simulink model "wall_plumbing"  (R2017b)
settings: Solver=VariableStepAuto  StartTime=0.0  StopTime=tf  RelTol=1e-3  AbsTol=1e-3  EnableMultiTasking=on
values from neighbouring files (symbols this model uses):
  cistern_diam = 100    [plumbing_variables.m]
  cistern_inlet_diam = 2    [plumbing_variables.m]
  cistern_outlet_diam = 2    [plumbing_variables.m]
  swh_inlet_diam = 2    [plumbing_variables.m]
  swh_outlet_diam = 2    [plumbing_variables.m]
libraries: fl_lib x40, nesl_utility x28, sh_lib x10, simulink x2, SimscapeFluids_lib x1
settings Model: Creator=solan  LastModifiedBy=solan
settings SolverCC: ZeroCrossAlgorithm=Adaptive
settings DataIOCC: LimitDataPoints=on  MaxDataPoints=10000
settings OptimizationCC: LifeSpan=inf
settings DebuggingCC: AllowSymbolicDim=off  SFUnexpectedBacktrackingDiag=warning  SFNoUnconditionalDefaultTransitionDiag=warning  SFExecutionAtInitializationDiag=none
settings CodeAppCC: StateflowObjectComments=on
settings GRTTargetCC: TargetLangStandard=C89/C90 (ANSI)  GeneratePreprocessorConditionals=Disable all
settings ConfigComp: CovMetricSettings=dw  CovHtmlReporting=on  CovSaveCumulativeToWorkspaceVar=on  CovSaveSingleToWorkspaceVar=on  CovExternalEMLEnable=off  CovSFcnEnable=off
settings SimscapeCC: SimscapeLogType=all  SimscapeLogSimulationStatistics=on  SimscapeLogOpenViewer=on  SimscapeLogDataHistory=10000

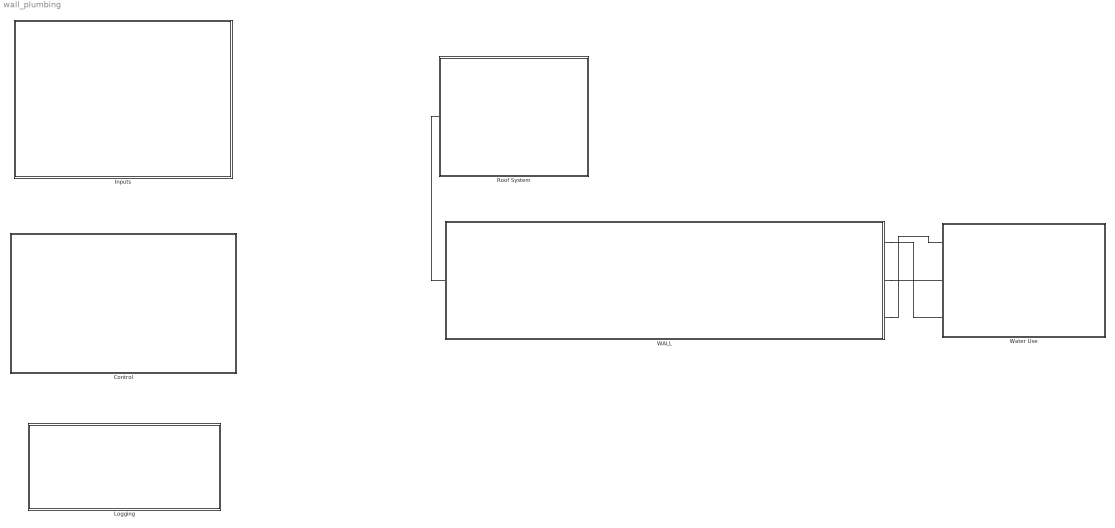
== system wall_plumbing ==
  Control : Subsystem
  Inputs : Subsystem
  Logging : Subsystem
  Roof System : Subsystem
  WALL : Subsystem
  Water Use : Subsystem
  connections:
  WALL/RConn2 -- Water Use/LConn3
  WALL/RConn1 -- Water Use/LConn2
  Roof System/LConn1 -- WALL/LConn1
  WALL/RConn3 -- Water Use/LConn1

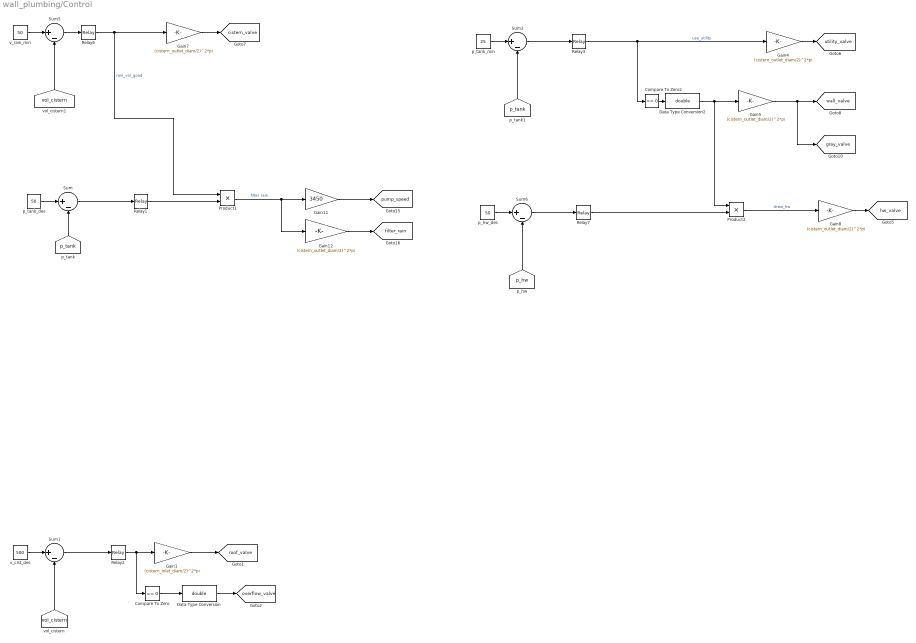
== system wall_plumbing/Control ==
  Compare To Zero : simulink/Logic and Bit Operations/Compare To Zero  relop===  OutDataTypeStr=boolean
  Compare To Zero2 : simulink/Logic and Bit Operations/Compare To Zero  relop===  OutDataTypeStr=boolean
  Data Type Conversion : DataTypeConversion  OutDataTypeStr=double
  Data Type Conversion2 : DataTypeConversion  OutDataTypeStr=double
  Gain1 : Gain  Gain=(cistern_inlet_diam/2)^2*pi
  Gain11 : Gain  Gain=3450
  Gain{4..5,7..8,12} (5 alike) : Gain  Gain=(cistern_outlet_diam/2)^2*pi
  Product1 : Product
  Product2 : Product
  Relay1 : Relay  OnSwitchValue=10  OffSwitchValue=-10
  Relay2 : Relay  OnSwitchValue=25  OffSwitchValue=-25
  Relay3 : Relay  OnSwitchValue=4  OffSwitchValue=-20
  Relay6 : Relay  OnSwitchValue=5  OffSwitchValue=-50  OnOutputValue=0  OffOutputValue=1
  Relay7 : Relay  OnSwitchValue=10  OffSwitchValue=-10
  Sum{,1..2,5..6} (5 alike) : Sum  Inputs=|+-
  p_hw_des : Constant  Value=50
  p_tank_des : Constant  Value=50
  p_tank_min : Constant  Value=25
  v_cist_des : Constant  Value=500
  v_rain_min : Constant  Value=50
  tag scope: cistern_valve=global, filter_rain=global, gray_valve=global, hw_valve=global, overflow_valve=global, pump_speed=global, roof_valve=global, utility_valve=global, wall_valve=global
  wires:
  Gain4/1 -> [utility_valve]
  Sum1/1 -> Relay2/1
  Relay3/1 -> Compare To Zero2/1, Gain4/1  "use_utility"
  Gain1/1 -> [roof_valve]
  v_cist_des/1 -> Sum1/1
  Data Type Conversion2/1 -> Product2/1, Gain5/1
  [vol_cistern] -> Sum1/2
  Sum/1 -> Relay1/1
  Gain5/1 -> [gray_valve], [wall_valve]
  [vol_cistern] -> Sum5/2
  Gain12/1 -> [filter_rain]
  [p_tank] -> Sum2/2
  Gain8/1 -> [hw_valve]
  p_tank_min/1 -> Sum2/1
  Relay1/1 -> Product1/2
  p_tank_des/1 -> Sum/1
  [p_tank] -> Sum/2
  Compare To Zero2/1 -> Data Type Conversion2/1
  Gain11/1 -> [pump_speed]
  Sum5/1 -> Relay6/1
  Sum6/1 -> Relay7/1
  Compare To Zero/1 -> Data Type Conversion/1
  p_hw_des/1 -> Sum6/1
  Gain7/1 -> [cistern_valve]
  [p_hw] -> Sum6/2
  Relay2/1 -> Compare To Zero/1, Gain1/1
  v_rain_min/1 -> Sum5/1
  Data Type Conversion/1 -> [overflow_valve]
  Relay6/1 -> Product1/1, Gain7/1  "rain_vol_good"
  Sum2/1 -> Relay3/1
  Product1/1 -> Gain12/1, Gain11/1  "filter rain"
  Relay7/1 -> Product2/2
  Product2/1 -> Gain8/1  "draw_hw"

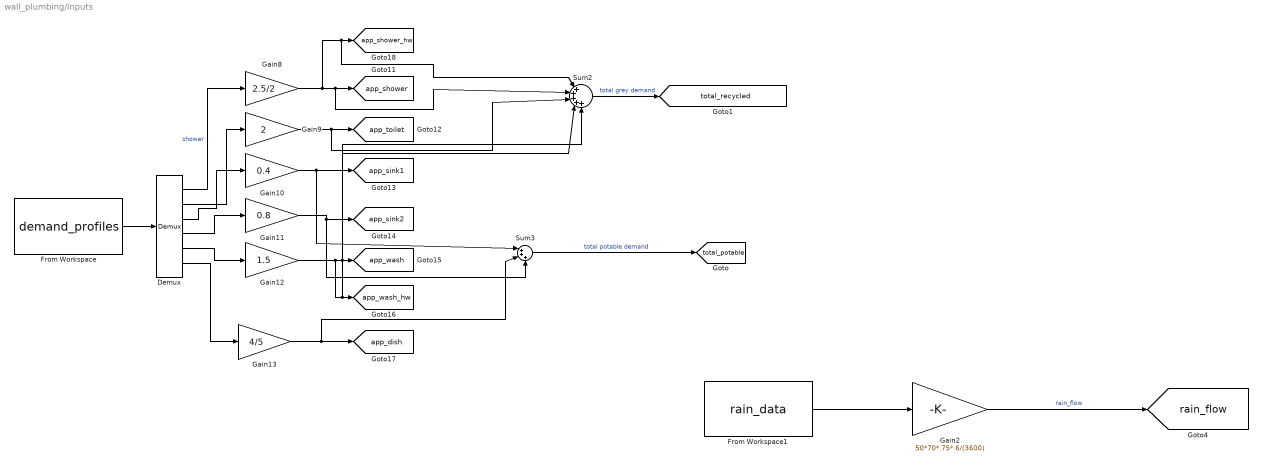
== system wall_plumbing/Inputs ==
  Demux : Demux  Outputs=6
  From Workspace : FromWorkspace  VariableName=demand_profiles  SampleTime=60
  From Workspace1 : FromWorkspace  VariableName=rain_data  SampleTime=0  Interpolate=off  OutputAfterFinalValue=Setting to zero
  Gain10 : Gain  Gain=0.4
  Gain11 : Gain  Gain=0.8
  Gain12 : Gain  Gain=1.5
  Gain13 : Gain  Gain=4/5
  Gain2 : Gain  Gain=50*70*.75*.6/(3600)
  Gain8 : Gain  Gain=2.5/2
  Gain9 : Gain  Gain=2
  Sum2 : Sum  Inputs=|+++++
  Sum3 : Sum  Inputs=|+++
  tag scope: app_dish=global, app_shower=global, app_shower_hw=global, app_sink1=global, app_sink2=global, app_toilet=global, app_wash=global, app_wash_hw=global, rain_flow=global, total_potable=global, total_recycled=global
  wires:
  From Workspace/1 -> Demux/1
  Demux/6 -> Gain13/1
  Gain2/1 -> [rain_flow]  "rain_flow"
  Gain9/1 -> Sum2/3, [app_toilet]
  Demux/4 -> Gain11/1
  Gain11/1 -> Sum3/3, [app_sink2]
  Demux/3 -> Gain10/1
  From Workspace1/1 -> Gain2/1
  Gain8/1 -> Sum2/1, [app_shower_hw], Sum2/2, [app_shower]
  Gain10/1 -> Sum3/1, [app_sink1]
  Demux/5 -> Gain12/1
  Demux/1 -> Gain8/1  "shower"
  Gain12/1 -> Sum2/5, [app_wash_hw], Sum2/4, [app_wash]
  Demux/2 -> Gain9/1
  Gain13/1 -> Sum3/2, [app_dish]
  Sum2/1 -> [total_recycled]  "total grey demand"
  Sum3/1 -> [total_potable]  "total potable demand"

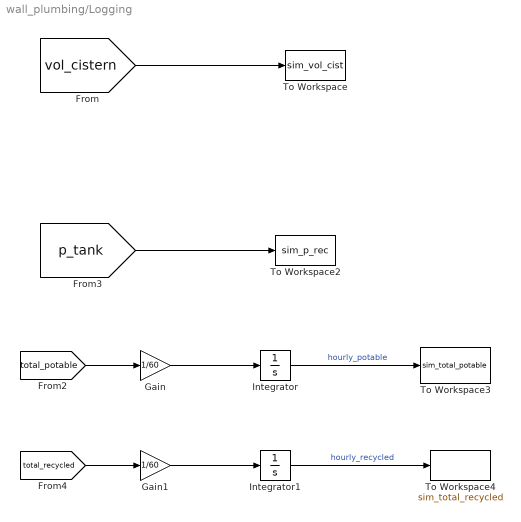
== system wall_plumbing/Logging ==
  Gain : Gain  Gain=1/60
  Gain1 : Gain  Gain=1/60
  Integrator : Integrator
  Integrator1 : Integrator
  To Workspace : ToWorkspace  VariableName=sim_vol_cist  SaveFormat=Timeseries  SampleTime=3600
  To Workspace2 : ToWorkspace  VariableName=sim_p_rec  SaveFormat=Timeseries  SampleTime=3600
  To Workspace3 : ToWorkspace  VariableName=sim_total_potable  SaveFormat=Timeseries  SampleTime=3600
  To Workspace4 : ToWorkspace  VariableName=sim_total_recycled  SaveFormat=Timeseries  SampleTime=3600
  wires:
  [vol_cistern] -> To Workspace/1
  [p_tank] -> To Workspace2/1
  [total_potable] -> Gain/1
  [total_recycled] -> Gain1/1
  Integrator1/1 -> To Workspace4/1  "hourly_recycled"
  Integrator/1 -> To Workspace3/1  "hourly_potable"
  Gain/1 -> Integrator/1
  Gain1/1 -> Integrator1/1

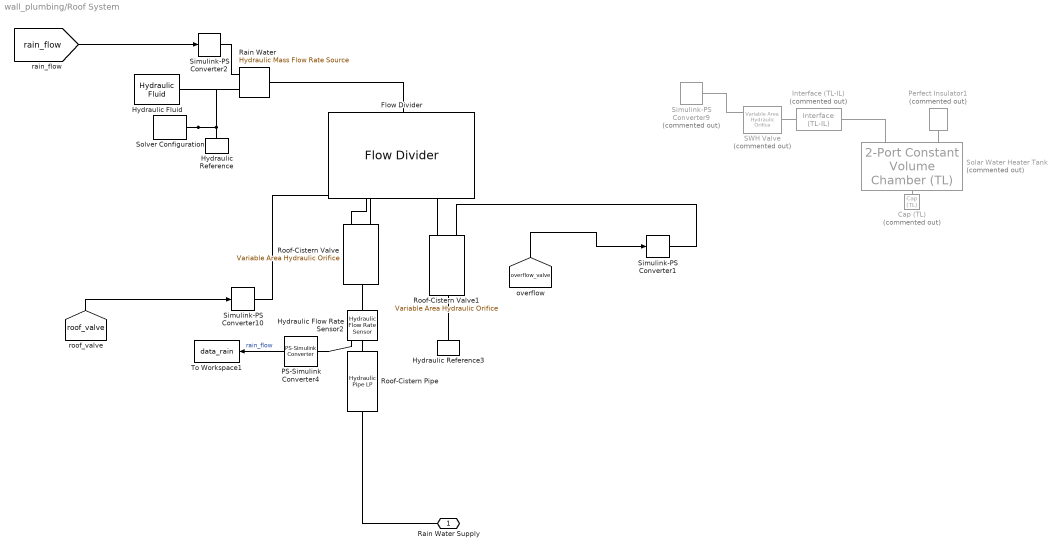
== system wall_plumbing/Roof System ==
  Cap (TL) : fl_lib/Thermal Liquid/Elements/Cap (TL)  Commented=on  p_specify=off  p_priority=None  p=0.101325 MPa  p_nominal_specify=off  p_nominal_unit=MPa  p_nominal_value=1  T_specify=off  T_priority=None  T=293.15 K  T_nominal_specify=off  T_nominal_unit=K  T_nominal_value=1
      settings: SourceProductName=Simscape  SourceProductBaseCode=SS
  Flow Divider : sh_lib/Valves/Flow Control Valves/Flow Divider  area_A=1e-4 m^2  area_B=1e-4 m^2  C_d_A=0.7  C_d_B=0.7  lam_spec=1  B_lam_A=0.999  B_lam_B=0.999  Re_cr_A=10  Re_cr_B=10  orifice_d=0.005 m  orifice_numb=4  C_d_or=0.65  init_A=0.0025 m  init_B=0.0025 m  leak_area=1e-9 m^2  lam_spec_or=1  B_lam_or_A=0.999  B_lam_or_B=0.999  Re_cr_or_A=10  Re_cr_or_B=10  area_sc=1.6e-4 m^2  stroke=0.005 m  spring_rate=1e3 N/m  damping=150 N/(m/s)  stop_coefficient=1e12 s*N/m^2
      settings: SourceProductName=Simscape Fluids  SourceProductBaseCode=SH
  Hydraulic Flow Rate Sensor2 : fl_lib/Hydraulic/Hydraulic Sensors/Hydraulic Flow Rate Sensor
      settings: SourceProductName=Simscape
  Hydraulic Fluid : sh_lib/Hydraulic Utilities/Hydraulic Fluid  DataSource=1  SelFluid=24  SysTemp=15  TrapAir=0.005  ViscDerFactor=1  range_error=2
      settings: SourceProductName=Simscape Fluids
  Hydraulic Reference : fl_lib/Hydraulic/Hydraulic Elements/Hydraulic Reference
      settings: SourceProductName=Foundation Library
  Hydraulic Reference3 : fl_lib/Hydraulic/Hydraulic Elements/Hydraulic Reference
      settings: SourceProductName=Foundation Library
  Interface (TL-IL) : SimscapeFluids_lib/Fluid Network Interfaces/Interface (TL-IL)  Commented=on  T_B=293.15 K  area=0.01 m^2
      settings: SourceProductName=Simscape Fluids  SourceProductBaseCode=SH
  PS-Simulink Converter4 : nesl_utility/PS-Simulink Converter  PhysicalDomain=network_engine_domain  SubClassName=ps_output  LeftPortType=input  RightPortType=output  PseudoPeriodic=off  Frequencies=[]  Unit=gal/s  AffineConversion=off
  Perfect Insulator1 : fl_lib/Thermal/Thermal Elements/Perfect Insulator  Commented=on  T_specify=off  T_priority=None  T=0 K  T_nominal_specify=off  T_nominal_unit=K  T_nominal_value=1
      settings: SourceProductName=Simscape
  Rain Water : fl_lib/Hydraulic/Hydraulic Sources/Hydraulic Mass Flow Rate Source
      settings: SourceProductName=Simscape  SourceProductBaseCode=SS
  Roof-Cistern Pipe : sh_lib/Low-Pressure Blocks/Hydraulic Pipe LP  cs_type=1  d_in=cistern_inlet_diam in  area=1e-4 m^2  D_h=1.12e-2 m  s_factor=64  length=roof_cistern_pipe_length ft  length_ad=1 m  roughness=15e-6 m  Re_lam=2000  Re_turb=4000  elevation_A=roof_height ft  elevation_B=cistern_inlet_height ft  g=9.80665 m/s^2  wall_type=1  pr_r_coef=2e-12 m/Pa  time_const=0.01 s  k_sh=1.4  p0=0 Pa
      settings: SourceProductName=Simscape Fluids  SourceProductBaseCode=SH
  Roof-Cistern Valve : fl_lib/Hydraulic/Hydraulic Elements/Variable Area Hydraulic Orifice  C_d=0.7  min_area=1e-12 m^2  lam_spec=1  B_lam=0.999  Re_cr=12  q_specify=off  q_priority=None  q=0.001 m^3/s  q_nominal_specify=off  q_nominal_unit=m^3/s  q_nominal_value=1  p_specify=off  p_priority=None  p=0 Pa  p_nominal_specify=off  p_nominal_unit=Pa  p_nominal_value=1
      settings: SourceProductName=Simscape  SourceProductBaseCode=SS
  Roof-Cistern Valve1 : fl_lib/Hydraulic/Hydraulic Elements/Variable Area Hydraulic Orifice  C_d=0.7  min_area=1e-12 m^2  lam_spec=1  B_lam=0.999  Re_cr=12  q_specify=off  q_priority=None  q=0.001 m^3/s  q_nominal_specify=off  q_nominal_unit=m^3/s  q_nominal_value=1  p_specify=off  p_priority=None  p=0 Pa  p_nominal_specify=off  p_nominal_unit=Pa  p_nominal_value=1
      settings: SourceProductName=Simscape  SourceProductBaseCode=SS
  SWH Valve : fl_lib/Hydraulic/Hydraulic Elements/Variable Area Hydraulic Orifice  Commented=on  C_d=0.7  min_area=1e-12 m^2  lam_spec=1  B_lam=0.999  Re_cr=12  q_specify=off  q_priority=None  q=0.001 m^3/s  q_nominal_specify=off  q_nominal_unit=m^3/s  q_nominal_value=1  p_specify=off  p_priority=None  p=0 Pa  p_nominal_specify=off  p_nominal_unit=Pa  p_nominal_value=1
      settings: SourceProductName=Simscape  SourceProductBaseCode=SS
  Simulink-PS Converter1 : nesl_utility/Simulink-PS Converter  PhysicalDomain=network_engine_domain  SubClassName=ps_input  LeftPortType=input  RightPortType=output  PseudoPeriodic=off  Frequencies=[]  NoiseDistribution=none  NoiseParameters=[]  Unit=1  AffineConversion=off  FilteringAndDerivatives=zero  SimscapeFilterOrder=1  InputFilterTimeConstant=0.001  UdotUserProvided=1
  Simulink-PS Converter10 : nesl_utility/Simulink-PS Converter  PhysicalDomain=network_engine_domain  SubClassName=ps_input  LeftPortType=input  RightPortType=output  PseudoPeriodic=off  Frequencies=[]  NoiseDistribution=none  NoiseParameters=[]  Unit=in^2  AffineConversion=off  FilteringAndDerivatives=zero  SimscapeFilterOrder=1  InputFilterTimeConstant=0.001  UdotUserProvided=1
  Simulink-PS Converter2 : nesl_utility/Simulink-PS Converter  PhysicalDomain=network_engine_domain  SubClassName=ps_input  LeftPortType=input  RightPortType=output  PseudoPeriodic=off  Frequencies=[]  NoiseDistribution=none  NoiseParameters=[]  Unit=kg/s  AffineConversion=off  FilteringAndDerivatives=zero  SimscapeFilterOrder=1  InputFilterTimeConstant=0.001  UdotUserProvided=1
  Simulink-PS Converter9 : nesl_utility/Simulink-PS Converter  Commented=on  PhysicalDomain=network_engine_domain  SubClassName=ps_input  LeftPortType=input  RightPortType=output  PseudoPeriodic=off  Frequencies=[]  NoiseDistribution=none  NoiseParameters=[]  Unit=1  AffineConversion=off  FilteringAndDerivatives=zero  SimscapeFilterOrder=1  InputFilterTimeConstant=0.001  UdotUserProvided=1
  Solar Water Heater Tank : fl_lib/Thermal Liquid/Elements/2-Port Constant Volume Chamber (TL)  Commented=on  volume=swh_volume gal  area_A=3.14*(swh_inlet_diam/2)^2 in^2  area_B=3.14*(swh_outlet_diam/2)^2 in^2  p_chamber_specify=off  p_chamber_priority=High  p_chamber=0.101325 MPa  p_chamber_nominal_specify=off  p_chamber_nominal_unit=MPa  p_chamber_nominal_value=1  T_chamber_specify=off  T_chamber_priority=High  T_chamber=293.15 K  T_chamber_nominal_specify=off  T_chamber_nominal_unit=K  T_chamber_nominal_value=1  u_chamber_specify=off  u_chamber_priority=None  u_chamber=83.90600000000001 kJ/kg  u_chamber_nominal_specify=off  u_chamber_nominal_unit=kJ/kg  u_chamber_nominal_value=1  rho_specify=off  rho_priority=None  rho=998.21 kg/m^3  rho_nominal_specify=off  rho_nominal_unit=kg/m^3  rho_nominal_value=1
      settings: SourceProductName=Simscape  SourceProductBaseCode=SS
  Solver Configuration : nesl_utility/Solver Configuration  PhysicalDomain=network_engine_domain  SubClassName=solver  LeftPortType=input  RightPortType=generic  Accelerate=off  Tones=[]  Harmonics=[]  SimulateNoise=off  Profile=off  UseLocalSampling=off  EnableSwitchedLinearOptims=on  FrequencyDomain=off  UseCCode=off  RelTol=0.001  AbsTol=1e-06  MinStep=1e-09  ToWorkspace=off  RevertToSquareIcSolve=off  NumHomotopyIterations=100  PhasorMode=off  PhasorModeNumHarmonics=1  DoDC=off  ResidualTolerance=1e-09  UseLocalSolver=off  LocalSolverChoice=NE_BACKWARD_EULER_ADVANCER  LocalSolverSampleTime=0.001  DoFixedCost=off  MaxNonlinIter=3  MaxModeIter=2  LinearAlgebra=Sparse  DelaysMemoryBudget=1024  AutomaticFiltering=on  FilteringTimeConstant=0.001
  To Workspace1 : ToWorkspace  VariableName=data_rain  SaveFormat=Timeseries  SampleTime=-1
  Rain Water Supply : PMIOPort  Port=1  Side=Left
  wires:
  [rain_flow] -> Simulink-PS Converter2/1
  [roof_valve] -> Simulink-PS Converter10/1
  [overflow_valve] -> Simulink-PS Converter1/1
  PS-Simulink Converter4/1 -> To Workspace1/1  "rain_flow"
  connections:
  Solver Configuration/RConn1 -- Rain Water/RConn2 -- Hydraulic Fluid/RConn1 -- Hydraulic Reference/LConn1
  SWH Valve/RConn1 -- Interface (TL-IL)/RConn1
  Interface (TL-IL)/LConn1 -- Solar Water Heater Tank/LConn1
  Simulink-PS Converter2/RConn1 -- Rain Water/RConn1
  Cap (TL)/LConn1 -- Solar Water Heater Tank/RConn1
  Perfect Insulator1/LConn1 -- Solar Water Heater Tank/LConn2
  Simulink-PS Converter9/RConn1 -- SWH Valve/LConn1
  Simulink-PS Converter10/RConn1 -- Roof-Cistern Valve/LConn1
  Flow Divider/RConn2 -- Roof-Cistern Valve/LConn2
  Hydraulic Reference3/LConn1 -- Roof-Cistern Valve1/RConn1
  Roof-Cistern Valve1/LConn2 -- Flow Divider/RConn1
  Simulink-PS Converter1/RConn1 -- Roof-Cistern Valve1/LConn1
  Rain Water/LConn1 -- Flow Divider/LConn1
  PS-Simulink Converter4/LConn1 -- Hydraulic Flow Rate Sensor2/RConn1
  Hydraulic Flow Rate Sensor2/LConn1 -- Roof-Cistern Valve/RConn1
  Roof-Cistern Pipe/LConn1 -- Hydraulic Flow Rate Sensor2/RConn2
  Roof-Cistern Pipe/RConn1 -- Rain Water Supply/RConn1

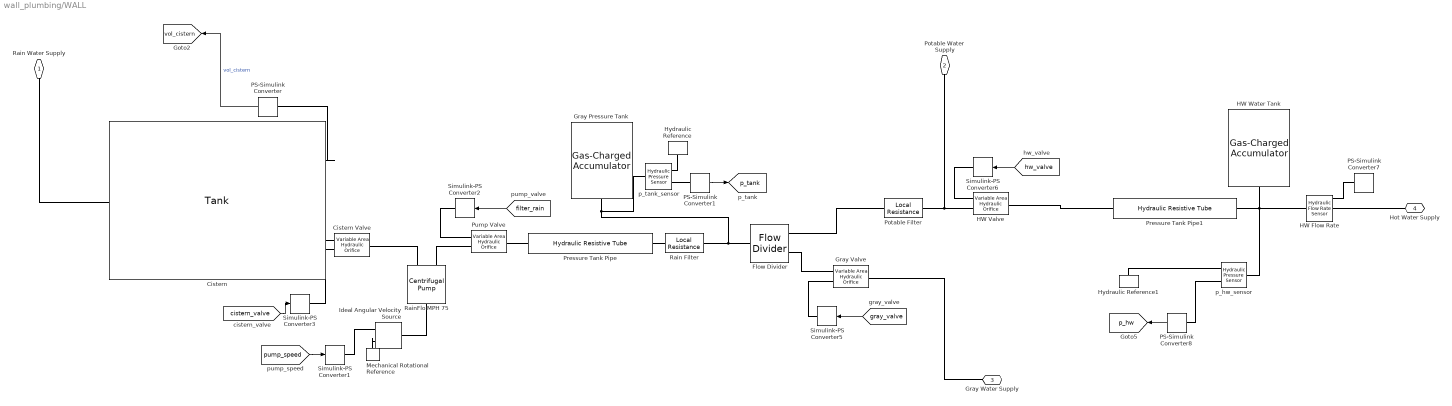
== system wall_plumbing/WALL ==
  Cistern : sh_lib/Low-Pressure Blocks/Tank  press=0 Pa  level_spec=1  tank_area=3.14*(cistern_diam/2)^2 in^2  fluid_volume_tab=[0, .0028, .0065, .0114, .0176, .0252, .0344, .0436, .0512, .0574, .0623, .066, .0688, .0707, .072, .0727] m^3  fluid_level_tab=[0, .02, .04, .06, .08, .1, .12, .14, .16, .18, .2, .22, .24, .26, .28, .3] m  interp_method=1  extrap_method=1  pipe_diam=0.02 m  loss_coeff=1.2  g=9.80665 m/s^2  min_level=1e-3 m  fluid_level_check=0  volume_specify=on  volume_priority=High  volume=480 gal  volume_nominal_specify=off  volume_nominal_unit=l  volume_nominal_value=1  level_specify=off  level_priority=None  level=0.025 m  level_nominal_specify=off  level_nominal_unit=m  level_nominal_value=1  pipe_diam_A=cistern_outlet_diam in  loss_coeff_A=1.2  height_B=cistern_inlet_height ft  pipe_diam_B=cistern_inlet_diam in  loss_coeff_B=1.2  height_C=0.8 m  pipe_diam_C=0.02 m  loss_coeff_C=1.2
      settings: SourceProductName=Simscape Fluids  SourceProductBaseCode=SH
  Cistern Valve : fl_lib/Hydraulic/Hydraulic Elements/Variable Area Hydraulic Orifice  C_d=0.7  min_area=1e-12 m^2  lam_spec=1  B_lam=0.999  Re_cr=12  q_specify=off  q_priority=None  q=0.001 m^3/s  q_nominal_specify=off  q_nominal_unit=m^3/s  q_nominal_value=1  p_specify=off  p_priority=None  p=0 Pa  p_nominal_specify=off  p_nominal_unit=Pa  p_nominal_value=1
      settings: SourceProductName=Simscape  SourceProductBaseCode=SS
  Flow Divider : sh_lib/Valves/Flow Control Valves/Flow Divider  area_A=pi in^2  area_B=pi in^2  C_d_A=0.7  C_d_B=0.7  lam_spec=1  B_lam_A=0.999  B_lam_B=0.999  Re_cr_A=10  Re_cr_B=10  orifice_d=0.005 m  orifice_numb=4  C_d_or=0.65  init_A=0.0025 m  init_B=0.0025 m  leak_area=1e-9 m^2  lam_spec_or=1  B_lam_or_A=0.999  B_lam_or_B=0.999  Re_cr_or_A=10  Re_cr_or_B=10  area_sc=1.6e-4 m^2  stroke=0.005 m  spring_rate=1e3 N/m  damping=150 N/(m/s)  stop_coefficient=1e12 s*N/m^2
      settings: SourceProductName=Simscape Fluids  SourceProductBaseCode=SH
  Gray Pressure Tank : sh_lib/Accumulators/Gas-Charged Accumulator  capacity=140/1.5 gal  dead_volume=23/1.5 gal  pr_preload=10 psi  k_sh=1.4  stiff_coeff=1e10 Pa/m^3  penetr_coeff=1e10 s*Pa/m^6  flow_rate_specify=off  flow_rate_priority=None  flow_rate=0.005 m^3/s  flow_rate_nominal_specify=off  flow_rate_nominal_unit=m^3/s  flow_rate_nominal_value=1  liquid_volume_specify=off  liquid_volume_priority=High  liquid_volume=80/1.5 m^3  liquid_volume_nominal_specify=off  liquid_volume_nominal_unit=m^3  liquid_volume_nominal_value=1  liquid_pressure_specify=off  liquid_pressure_priority=None  liquid_pressure=1.01325e+5 Pa  liquid_pressure_nominal_specify=off  liquid_pressure_nominal_unit=Pa  liquid_pressure_nominal_value=1
      settings: SourceProductName=Simscape Fluids  SourceProductBaseCode=SH
  Gray Valve : fl_lib/Hydraulic/Hydraulic Elements/Variable Area Hydraulic Orifice  C_d=0.7  min_area=1e-12 m^2  lam_spec=1  B_lam=0.999  Re_cr=12  q_specify=off  q_priority=None  q=0.001 m^3/s  q_nominal_specify=off  q_nominal_unit=m^3/s  q_nominal_value=1  p_specify=off  p_priority=None  p=0 Pa  p_nominal_specify=off  p_nominal_unit=Pa  p_nominal_value=1
      settings: SourceProductName=Simscape  SourceProductBaseCode=SS
  HW Flow Rate : fl_lib/Hydraulic/Hydraulic Sensors/Hydraulic Flow Rate Sensor
      settings: SourceProductName=Simscape
  HW Valve : fl_lib/Hydraulic/Hydraulic Elements/Variable Area Hydraulic Orifice  C_d=0.7  min_area=1e-12 m^2  lam_spec=1  B_lam=0.999  Re_cr=12  q_specify=off  q_priority=None  q=0.001 m^3/s  q_nominal_specify=off  q_nominal_unit=m^3/s  q_nominal_value=1  p_specify=off  p_priority=None  p=0 Pa  p_nominal_specify=off  p_nominal_unit=Pa  p_nominal_value=1
      settings: SourceProductName=Simscape  SourceProductBaseCode=SS
  HW Water Tank : sh_lib/Accumulators/Gas-Charged Accumulator  capacity=140/2 gal  dead_volume=23/2 gal  pr_preload=10 psi  k_sh=1.4  stiff_coeff=1e10 Pa/m^3  penetr_coeff=1e10 s*Pa/m^6  flow_rate_specify=off  flow_rate_priority=None  flow_rate=0.005 m^3/s  flow_rate_nominal_specify=off  flow_rate_nominal_unit=m^3/s  flow_rate_nominal_value=1  liquid_volume_specify=on  liquid_volume_priority=High  liquid_volume=40 gal  liquid_volume_nominal_specify=off  liquid_volume_nominal_unit=m^3  liquid_volume_nominal_value=1  liquid_pressure_specify=off  liquid_pressure_priority=None  liquid_pressure=1.01325e+5 Pa  liquid_pressure_nominal_specify=off  liquid_pressure_nominal_unit=Pa  liquid_pressure_nominal_value=1
      settings: SourceProductName=Simscape Fluids  SourceProductBaseCode=SH
  Hydraulic Reference : fl_lib/Hydraulic/Hydraulic Elements/Hydraulic Reference
      settings: SourceProductName=Foundation Library
  Hydraulic Reference1 : fl_lib/Hydraulic/Hydraulic Elements/Hydraulic Reference
      settings: SourceProductName=Foundation Library
  Ideal Angular Velocity Source : fl_lib/Mechanical/Mechanical Sources/Ideal Angular Velocity Source
  Mechanical Rotational Reference : fl_lib/Mechanical/Rotational Elements/Mechanical Rotational Reference
  PS-Simulink Converter : nesl_utility/PS-Simulink Converter  PhysicalDomain=network_engine_domain  SubClassName=ps_output  LeftPortType=input  RightPortType=output  PseudoPeriodic=off  Frequencies=[]  Unit=gal  AffineConversion=off
  PS-Simulink Converter1 : nesl_utility/PS-Simulink Converter  PhysicalDomain=network_engine_domain  SubClassName=ps_output  LeftPortType=input  RightPortType=output  PseudoPeriodic=off  Frequencies=[]  Unit=psi  AffineConversion=off
  PS-Simulink Converter7 : nesl_utility/PS-Simulink Converter  PhysicalDomain=network_engine_domain  SubClassName=ps_output  LeftPortType=input  RightPortType=output  PseudoPeriodic=off  Frequencies=[]  Unit=gal/min  AffineConversion=off
  PS-Simulink Converter8 : nesl_utility/PS-Simulink Converter  PhysicalDomain=network_engine_domain  SubClassName=ps_output  LeftPortType=input  RightPortType=output  PseudoPeriodic=off  Frequencies=[]  Unit=psi  AffineConversion=off
  Potable Filter : sh_lib/Local Hydraulic Resistances/Local Resistance  area=1e-4 m^2  mdl_type=1  kp_d=2  kp_r=2  lam_spec=1  B_lam=0.999  Re_cr=150  Re_vec=[-4000, -3000, -2000, -1000, -500, -200, -100, -50, -40, -30, -20, -15, -10, 10, 20, 30, 40, 50, 100, 200, 500, 1000, 2000, 4000, 5000, 10000]  loss_coeff_vec=[.25, .3, .65, .9, .65, .75, .9, 1.15, 1.35, 1.65, 2.3, 2.8, 3.1, 5, 2.7, 1.8, 1.46, 1.3, .9, .65, .42, .3, .2, .4, .42, .25]  interp_method=2  extrap_method=2  flow_rate_specify=off  flow_rate_priority=None  flow_rate=0 m^3/s  flow_rate_nominal_specify=off  flow_rate_nominal_unit=m^3/s  flow_rate_nominal_value=1  pressure_drop_specify=off  pressure_drop_priority=None  pressure_drop=0 Pa  pressure_drop_nominal_specify=off  pressure_drop_nominal_unit=Pa  pressure_drop_nominal_value=1
      settings: SourceProductName=Simscape Fluids  SourceProductBaseCode=SH
  Pressure Tank Pipe : fl_lib/Hydraulic/Hydraulic Elements/Hydraulic Resistive Tube  cs_type=1  d_in=2 in  area=1e-4 m^2  D_h=1.12e-2 m  s_factor=64  length=ptank_pipe_length ft  length_ad=1 m  roughness=15e-6 m  Re_lam=2000  Re_turb=4000  q_specify=off  q_priority=None  q=0.001 m^3/s  q_nominal_specify=off  q_nominal_unit=m^3/s  q_nominal_value=1  p_specify=off  p_priority=None  p=0 Pa  p_nominal_specify=off  p_nominal_unit=Pa  p_nominal_value=1
      settings: SourceProductName=Simscape  SourceProductBaseCode=SS
  Pressure Tank Pipe1 : fl_lib/Hydraulic/Hydraulic Elements/Hydraulic Resistive Tube  cs_type=1  d_in=1/4 in  area=1e-4 m^2  D_h=1.12e-2 m  s_factor=64  length=ptank_pipe_length ft  length_ad=1 m  roughness=15e-6 m  Re_lam=2000  Re_turb=4000  q_specify=off  q_priority=None  q=0.001 m^3/s  q_nominal_specify=off  q_nominal_unit=m^3/s  q_nominal_value=1  p_specify=off  p_priority=None  p=0 Pa  p_nominal_specify=off  p_nominal_unit=Pa  p_nominal_value=1
      settings: SourceProductName=Simscape  SourceProductBaseCode=SS
  Pump Valve : fl_lib/Hydraulic/Hydraulic Elements/Variable Area Hydraulic Orifice  C_d=0.7  min_area=1e-12 m^2  lam_spec=1  B_lam=0.999  Re_cr=12  q_specify=off  q_priority=None  q=0.001 m^3/s  q_nominal_specify=off  q_nominal_unit=m^3/s  q_nominal_value=1  p_specify=off  p_priority=None  p=0 Pa  p_nominal_specify=off  p_nominal_unit=Pa  p_nominal_value=1
      settings: SourceProductName=Simscape  SourceProductBaseCode=SS
  Rain Filter : sh_lib/Local Hydraulic Resistances/Local Resistance  area=1e-4 m^2  mdl_type=1  kp_d=2  kp_r=2  lam_spec=1  B_lam=0.999  Re_cr=150  Re_vec=[-4000, -3000, -2000, -1000, -500, -200, -100, -50, -40, -30, -20, -15, -10, 10, 20, 30, 40, 50, 100, 200, 500, 1000, 2000, 4000, 5000, 10000]  loss_coeff_vec=[.25, .3, .65, .9, .65, .75, .9, 1.15, 1.35, 1.65, 2.3, 2.8, 3.1, 5, 2.7, 1.8, 1.46, 1.3, .9, .65, .42, .3, .2, .4, .42, .25]  interp_method=2  extrap_method=2  flow_rate_specify=off  flow_rate_priority=None  flow_rate=0 m^3/s  flow_rate_nominal_specify=off  flow_rate_nominal_unit=m^3/s  flow_rate_nominal_value=1  pressure_drop_specify=off  pressure_drop_priority=None  pressure_drop=0 Pa  pressure_drop_nominal_specify=off  pressure_drop_nominal_unit=Pa  pressure_drop_nominal_value=1
      settings: SourceProductName=Simscape Fluids  SourceProductBaseCode=SH
  RainFlo MPH 75 : sh_lib/Pumps and Motors/Centrifugal Pump  mdl_type=2  c_1=326.8 Pa/(kg/m^3)  c_2=3.104e+4 Pa*s/kg  c_3=1.097e+7 Pa*s^2/(kg*m^3)  c_4=2.136e+5 Pa*s^2/(kg*m^3)  c_f=0.8  design_del=130 lpm  ref_velocity=3.45e+3 rpm  ref_density=940 kg/m^3  leak_resistance=1e+8 Pa/(m^3/s)  T_const=0.1 N*m  trq_press_coeff=1e-6 N*m/Pa  pump_del_1D=[0 6.5 9.2 11.7 14.0 15.8 17.0 18.8 20.2 21.4 22.7 24.0 25.0 26.2 ] gpm  press_diff_1D=[70 65 60 55 50 45 40 35 30 25 20 15 10 5.5 ] psi  pump_del_power_1D="[0 7.7 12.9 16.5  22.1 26.2 ] gpm"  power_1D="(0.75/1.7)*[0 7.8e-01   2.1   2.4   2.16   1.7] HP"  pump_del_2D=[ 0 50 100 150 200 250 300 350 ] lpm  pump_vel_2D=[ 3.2e+3 3.3e+3 3.4e+3 3.5e+3 ] rpm  press_diff_2D=[ 8.300000000000001 8.800000000000001 9.300000000000001 9.9; 7.8 8.300000000000001 8.800000000000001 9.4; 7.2 7.6 8.199999999999999 8.699999999999999; 6.5 7 7.5 8; 5.6 6.1 6.6 7.1; 4.7 5.2 5.7 6.2; 3.4 4 4.4 4.9; 2.3 2.7 3.4 3.6 ] bar  pump_del_power_2D=[ 0 50 100 150 200 250 300 350 ] lpm  power_2D=[ 1.223e+3 1.341e+3 1.467e+3 1.6e+3; 1.414e+3 1.551e+3 1.696e+3 1.85e+3; 1.636e+3 1.794e+3 1.962e+3 2.14e+3; 1.941e+3 2.129e+3 2.326e+3 2.54e+3; 2.224e+3 2.439e+3 2.66e+3 2.91e+3; 2.453e+3 2.691e+3 2.947e+3 3.21e+3; 2.757e+3 3.024e+3 3.307e+3 3.608e+3; 2.945e+3 3.23e+3 3.533e+3 3.854e+3 ] W  interp_method=1  extrap_method=1
      settings: SourceProductName=Simscape Fluids  SourceProductBaseCode=SH
  Simulink-PS Converter1 : nesl_utility/Simulink-PS Converter  PhysicalDomain=network_engine_domain  SubClassName=ps_input  LeftPortType=input  RightPortType=output  PseudoPeriodic=off  Frequencies=[]  NoiseDistribution=none  NoiseParameters=[]  Unit=rpm  AffineConversion=off  FilteringAndDerivatives=zero  SimscapeFilterOrder=1  InputFilterTimeConstant=0.001  UdotUserProvided=1
  Simulink-PS Converter{2..3,5..6} (4 alike) : nesl_utility/Simulink-PS Converter  PhysicalDomain=network_engine_domain  SubClassName=ps_input  LeftPortType=input  RightPortType=output  PseudoPeriodic=off  Frequencies=[]  NoiseDistribution=none  NoiseParameters=[]  Unit=in^2  AffineConversion=off  FilteringAndDerivatives=zero  SimscapeFilterOrder=1  InputFilterTimeConstant=0.001  UdotUserProvided=1
  p_hw_sensor : fl_lib/Hydraulic/Hydraulic Sensors/Hydraulic Pressure Sensor
      settings: SourceProductName=Simscape
  p_tank_sensor : fl_lib/Hydraulic/Hydraulic Sensors/Hydraulic Pressure Sensor
      settings: SourceProductName=Simscape
  Rain Water Supply : PMIOPort  Port=1  Side=Left
  Potable Water Supply : PMIOPort  Port=2  Side=Right
  Gray Water Supply : PMIOPort  Port=3  Side=Right
  Hot Water Supply : PMIOPort  Port=4  Side=Right
  tag scope: p_hw=global, p_tank=global, vol_cistern=global
  wires:
  PS-Simulink Converter/1 -> [vol_cistern]  "vol_cistern"
  PS-Simulink Converter1/1 -> [p_tank]
  [filter_rain] -> Simulink-PS Converter2/1
  [cistern_valve] -> Simulink-PS Converter3/1
  [pump_speed] -> Simulink-PS Converter1/1
  [gray_valve] -> Simulink-PS Converter5/1
  [hw_valve] -> Simulink-PS Converter6/1
  PS-Simulink Converter8/1 -> [p_hw]
  connections:
  Ideal Angular Velocity Source/LConn1 -- RainFlo MPH 75/LConn1
  Cistern/LConn1 -- Rain Water Supply/RConn1
  Gray Pressure Tank/RConn1 -- Rain Filter/RConn1 -- Flow Divider/LConn1 -- p_tank_sensor/LConn1
  Simulink-PS Converter1/RConn1 -- Ideal Angular Velocity Source/RConn1
  Mechanical Rotational Reference/LConn1 -- Ideal Angular Velocity Source/RConn2
  Cistern/RConn1 -- PS-Simulink Converter/LConn1
  Hydraulic Reference/LConn1 -- p_tank_sensor/RConn1
  PS-Simulink Converter1/LConn1 -- p_tank_sensor/RConn2
  RainFlo MPH 75/RConn1 -- Pump Valve/LConn2
  Pump Valve/LConn1 -- Simulink-PS Converter2/RConn1
  Cistern Valve/LConn2 -- Cistern/RConn2
  RainFlo MPH 75/RConn2 -- Cistern Valve/RConn1
  Simulink-PS Converter3/RConn1 -- Cistern Valve/LConn1
  Pressure Tank Pipe/LConn1 -- Pump Valve/RConn1
  Rain Filter/LConn1 -- Pressure Tank Pipe/RConn1
  Potable Filter/LConn1 -- Flow Divider/RConn1
  Flow Divider/RConn2 -- Gray Valve/LConn2
  Simulink-PS Converter5/RConn1 -- Gray Valve/LConn1
  Gray Water Supply/RConn1 -- Gray Valve/RConn1
  Potable Water Supply/RConn1 -- Potable Filter/RConn1 -- HW Valve/LConn2
  HW Valve/LConn1 -- Simulink-PS Converter6/RConn1
  HW Flow Rate/LConn1 -- HW Water Tank/RConn1 -- Pressure Tank Pipe1/RConn1 -- p_hw_sensor/LConn1
  PS-Simulink Converter7/LConn1 -- HW Flow Rate/RConn1
  PS-Simulink Converter8/LConn1 -- p_hw_sensor/RConn2
  Hot Water Supply/RConn1 -- HW Flow Rate/RConn2
  p_hw_sensor/RConn1 -- Hydraulic Reference1/LConn1
  HW Valve/RConn1 -- Pressure Tank Pipe1/LConn1

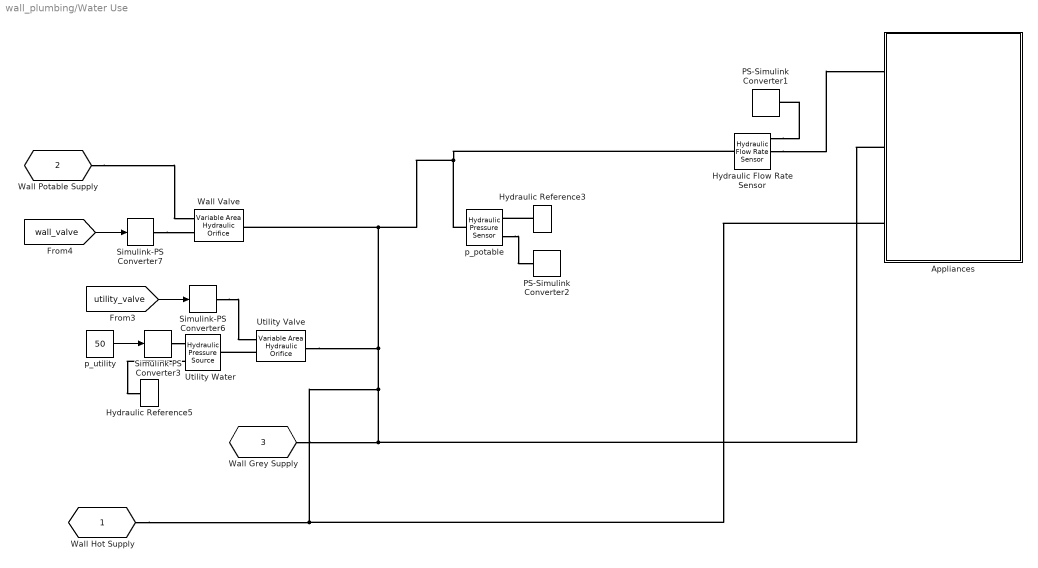
== system wall_plumbing/Water Use ==
  Appliances : Subsystem
  Hydraulic Flow Rate Sensor : fl_lib/Hydraulic/Hydraulic Sensors/Hydraulic Flow Rate Sensor
      settings: SourceProductName=Simscape
  Hydraulic Reference3 : fl_lib/Hydraulic/Hydraulic Elements/Hydraulic Reference
      settings: SourceProductName=Foundation Library
  Hydraulic Reference5 : fl_lib/Hydraulic/Hydraulic Elements/Hydraulic Reference
      settings: SourceProductName=Foundation Library
  PS-Simulink Converter1 : nesl_utility/PS-Simulink Converter  PhysicalDomain=network_engine_domain  SubClassName=ps_output  LeftPortType=input  RightPortType=output  PseudoPeriodic=off  Frequencies=[]  Unit=gal/s  AffineConversion=off
  PS-Simulink Converter2 : nesl_utility/PS-Simulink Converter  PhysicalDomain=network_engine_domain  SubClassName=ps_output  LeftPortType=input  RightPortType=output  PseudoPeriodic=off  Frequencies=[]  Unit=psi  AffineConversion=off
  Simulink-PS Converter3 : nesl_utility/Simulink-PS Converter  PhysicalDomain=network_engine_domain  SubClassName=ps_input  LeftPortType=input  RightPortType=output  PseudoPeriodic=off  Frequencies=[]  NoiseDistribution=none  NoiseParameters=[]  Unit=1  AffineConversion=off  FilteringAndDerivatives=zero  SimscapeFilterOrder=1  InputFilterTimeConstant=0.001  UdotUserProvided=1
  Simulink-PS Converter6 : nesl_utility/Simulink-PS Converter  PhysicalDomain=network_engine_domain  SubClassName=ps_input  LeftPortType=input  RightPortType=output  PseudoPeriodic=off  Frequencies=[]  NoiseDistribution=none  NoiseParameters=[]  Unit=in^2  AffineConversion=off  FilteringAndDerivatives=zero  SimscapeFilterOrder=1  InputFilterTimeConstant=0.001  UdotUserProvided=1
  Simulink-PS Converter7 : nesl_utility/Simulink-PS Converter  PhysicalDomain=network_engine_domain  SubClassName=ps_input  LeftPortType=input  RightPortType=output  PseudoPeriodic=off  Frequencies=[]  NoiseDistribution=none  NoiseParameters=[]  Unit=in^2  AffineConversion=off  FilteringAndDerivatives=zero  SimscapeFilterOrder=1  InputFilterTimeConstant=0.001  UdotUserProvided=1
  Utility Valve : fl_lib/Hydraulic/Hydraulic Elements/Variable Area Hydraulic Orifice  C_d=0.7  min_area=1e-12 m^2  lam_spec=1  B_lam=0.999  Re_cr=12  q_specify=off  q_priority=None  q=0.001 m^3/s  q_nominal_specify=off  q_nominal_unit=m^3/s  q_nominal_value=1  p_specify=off  p_priority=None  p=0 Pa  p_nominal_specify=off  p_nominal_unit=Pa  p_nominal_value=1
      settings: SourceProductName=Simscape  SourceProductBaseCode=SS
  Utility Water : fl_lib/Hydraulic/Hydraulic Sources/Hydraulic Pressure Source
      settings: SourceProductName=Simscape  SourceProductBaseCode=SS
  Wall Valve : fl_lib/Hydraulic/Hydraulic Elements/Variable Area Hydraulic Orifice  C_d=0.7  min_area=1e-12 m^2  lam_spec=1  B_lam=0.999  Re_cr=12  q_specify=off  q_priority=None  q=0.001 m^3/s  q_nominal_specify=off  q_nominal_unit=m^3/s  q_nominal_value=1  p_specify=off  p_priority=None  p=0 Pa  p_nominal_specify=off  p_nominal_unit=Pa  p_nominal_value=1
      settings: SourceProductName=Simscape  SourceProductBaseCode=SS
  p_potable : fl_lib/Hydraulic/Hydraulic Sensors/Hydraulic Pressure Sensor
      settings: SourceProductName=Simscape
  p_utility : Constant  Value=50
  Wall Hot Supply : PMIOPort  Port=1  Side=Left
  Wall Potable Supply : PMIOPort  Port=2  Side=Left
  Wall Grey Supply : PMIOPort  Port=3  Side=Left
  wires:
  [wall_valve] -> Simulink-PS Converter7/1
  [utility_valve] -> Simulink-PS Converter6/1
  p_utility/1 -> Simulink-PS Converter3/1
  connections:
  p_potable/RConn2 -- PS-Simulink Converter2/LConn1
  Simulink-PS Converter7/RConn1 -- Wall Valve/LConn1
  Hydraulic Flow Rate Sensor/LConn1 -- p_potable/LConn1 -- Appliances/LConn3 -- Wall Hot Supply/RConn1 -- Appliances/LConn2 -- Wall Grey Supply/RConn1 -- Utility Valve/RConn1 -- Wall Valve/RConn1
  Hydraulic Flow Rate Sensor/RConn1 -- PS-Simulink Converter1/LConn1
  Wall Potable Supply/RConn1 -- Wall Valve/LConn2
  Hydraulic Reference3/LConn1 -- p_potable/RConn1
  Hydraulic Flow Rate Sensor/RConn2 -- Appliances/LConn1
  Simulink-PS Converter6/RConn1 -- Utility Valve/LConn1
  Utility Valve/LConn2 -- Utility Water/LConn1
  Simulink-PS Converter3/RConn1 -- Utility Water/RConn1
  Utility Water/RConn2 -- Hydraulic Reference5/LConn1

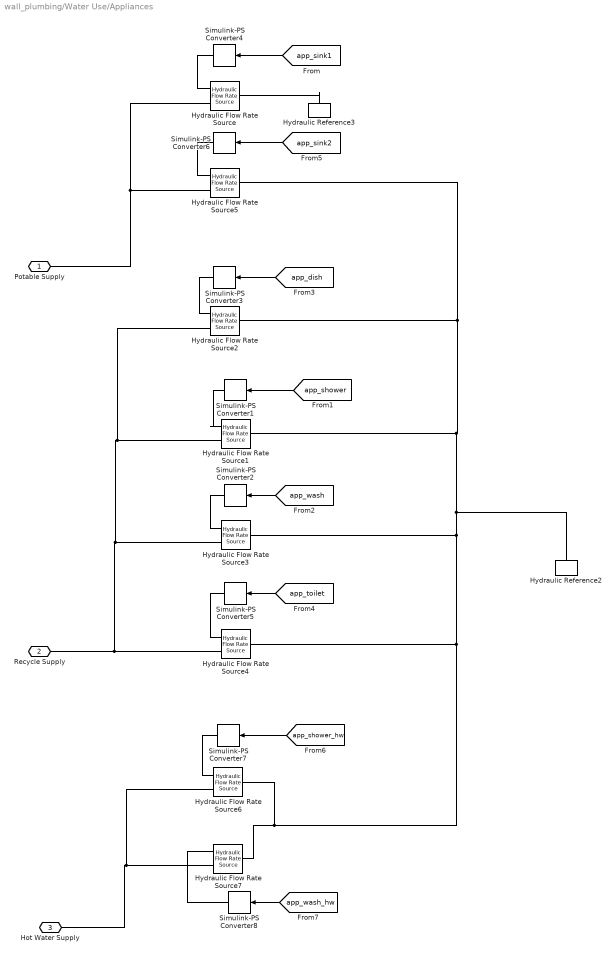
== system wall_plumbing/Water Use/Appliances ==
  Hydraulic Flow Rate Source{,1..7} (8 alike) : fl_lib/Hydraulic/Hydraulic Sources/Hydraulic Flow Rate Source
      settings: SourceProductName=Simscape  SourceProductBaseCode=SS
  Hydraulic Reference2 : fl_lib/Hydraulic/Hydraulic Elements/Hydraulic Reference
      settings: SourceProductName=Simscape
  Hydraulic Reference3 : fl_lib/Hydraulic/Hydraulic Elements/Hydraulic Reference
      settings: SourceProductName=Simscape
  Simulink-PS Converter{1..8} (8 alike) : nesl_utility/Simulink-PS Converter  PhysicalDomain=network_engine_domain  SubClassName=ps_input  LeftPortType=input  RightPortType=output  PseudoPeriodic=off  Frequencies=[]  NoiseDistribution=none  NoiseParameters=[]  Unit=gal/min  AffineConversion=off  FilteringAndDerivatives=zero  SimscapeFilterOrder=1  InputFilterTimeConstant=0.001  UdotUserProvided=1
  Potable Supply : PMIOPort  Port=1  Side=Left
  Recycle Supply : PMIOPort  Port=2  Side=Left
  Hot Water Supply : PMIOPort  Port=3  Side=Left
  wires:
  [app_wash_hw] -> Simulink-PS Converter8/1
  [app_shower] -> Simulink-PS Converter1/1
  [app_toilet] -> Simulink-PS Converter5/1
  [app_shower_hw] -> Simulink-PS Converter7/1
  [app_wash] -> Simulink-PS Converter2/1
  [app_dish] -> Simulink-PS Converter3/1
  [app_sink2] -> Simulink-PS Converter6/1
  [app_sink1] -> Simulink-PS Converter4/1
  connections:
  Hydraulic Flow Rate Source2/LConn1 -- Hydraulic Reference2/LConn1 -- Hydraulic Flow Rate Source4/LConn1 -- Hydraulic Flow Rate Source6/LConn1 -- Hydraulic Flow Rate Source7/LConn1 -- Hydraulic Flow Rate Source3/LConn1 -- Hydraulic Flow Rate Source1/LConn1 -- Hydraulic Flow Rate Source5/LConn1
  Hydraulic Flow Rate Source7/RConn2 -- Hot Water Supply/RConn1 -- Hydraulic Flow Rate Source6/RConn2
  Hydraulic Flow Rate Source/RConn2 -- Potable Supply/RConn1 -- Hydraulic Flow Rate Source5/RConn2
  Hydraulic Flow Rate Source4/RConn2 -- Recycle Supply/RConn1 -- Hydraulic Flow Rate Source2/RConn2 -- Hydraulic Flow Rate Source1/RConn2 -- Hydraulic Flow Rate Source3/RConn2
  Simulink-PS Converter7/RConn1 -- Hydraulic Flow Rate Source6/RConn1
  Hydraulic Flow Rate Source7/RConn1 -- Simulink-PS Converter8/RConn1
  Hydraulic Flow Rate Source1/RConn1 -- Simulink-PS Converter1/RConn1
  Hydraulic Flow Rate Source2/RConn1 -- Simulink-PS Converter3/RConn1
  Hydraulic Flow Rate Source3/RConn1 -- Simulink-PS Converter2/RConn1
  Hydraulic Flow Rate Source5/RConn1 -- Simulink-PS Converter6/RConn1
  Hydraulic Flow Rate Source/RConn1 -- Simulink-PS Converter4/RConn1
  Hydraulic Reference3/LConn1 -- Hydraulic Flow Rate Source/LConn1
  Hydraulic Flow Rate Source4/RConn1 -- Simulink-PS Converter5/RConn1
